simulink library "halin"  (R2021b)
settings: Solver=VariableStepAuto  StartTime=0.0  StopTime=10.0  RelTol=1e-3
undefined symbols (not defined in the file): KHAL_CAN1ABM1E2E_flg, KHAL_CAN1EPB1E2E_flg, KHAL_CAN1EPS1E2E_flg, KHAL_CAN1ESC1E2E_flg, KHAL_CAN1ESC5E2E_flg, KHAL_CAN3BMS1E2E_flg, KHAL_CAN3BMS6E2E_flg, KHAL_CAN3CCU1E2E_flg, KHAL_CAN3CCU2E2E_flg, KHAL_CAN3MCUNF1E2E_flg, KHAL_CAN3MCUNR1E2E_flg, KHAL_CAN3Shifter1E2E_flg, KHAL_CAN3Shifter2E2E_flg, KHAL_CAN6FCM2E2E_flg, KHAL_CAN6FCM4E2E_flg, TRUE
libraries: simulink x645, FVT_lib x212, hcu_lib x59
(part 18 of 23)

== system halin/HAL_IN/CAN1/EPS1/SASSpeedValid ==
  SAS_Speed_Valid : Inport
  UnitConverter : DataTypeConversion  OutDataTypeStr=uint8
  VHAL_SASSpeedValid_flg : Outport
  wires:
  UnitConverter/1 -> VHAL_SASSpeedValid_flg/1
  SAS_Speed_Valid/1 -> UnitConverter/1

== system halin/HAL_IN/CAN1/EPS1/SASV ==
  SAS_V : Inport
  UnitConverter : DataTypeConversion  OutDataTypeStr=uint8
  VHAL_SASV_flg : Outport
  wires:
  UnitConverter/1 -> VHAL_SASV_flg/1
  SAS_V/1 -> UnitConverter/1

== system halin/HAL_IN/CAN1/ESC1/ABSActive ==
  ABS_Active : Inport
  UnitConverter : DataTypeConversion  OutDataTypeStr=uint8
  VHAL_ABSActive_flg : Outport
  wires:
  UnitConverter/1 -> VHAL_ABSActive_flg/1
  ABS_Active/1 -> UnitConverter/1

== system halin/HAL_IN/CAN1/ESC1/ABSFailed ==
  ABS_Failed : Inport
  UnitConverter : DataTypeConversion  OutDataTypeStr=uint8
  VHAL_ABSFailed_flg : Outport
  wires:
  UnitConverter/1 -> VHAL_ABSFailed_flg/1
  ABS_Failed/1 -> UnitConverter/1

== system halin/HAL_IN/CAN1/ESC1/ABSWnlmpSta ==
  ABS_WnlmpSta : Inport
  UnitConverter : DataTypeConversion  OutDataTypeStr=uint8
  VHAL_ABSWnlmpSta_flg : Outport
  wires:
  UnitConverter/1 -> VHAL_ABSWnlmpSta_flg/1
  ABS_WnlmpSta/1 -> UnitConverter/1

== system halin/HAL_IN/CAN1/ESC1/AVHActive ==
  AVH_Active : Inport
  UnitConverter : DataTypeConversion  OutDataTypeStr=uint8
  VHAL_AVHActive_flg : Outport
  wires:
  UnitConverter/1 -> VHAL_AVHActive_flg/1
  AVH_Active/1 -> UnitConverter/1

== system halin/HAL_IN/CAN1/ESC1/AVHFailed ==
  AVH_Failed : Inport
  UnitConverter : DataTypeConversion  OutDataTypeStr=uint8
  VHAL_AVHFailed_flg : Outport
  wires:
  UnitConverter/1 -> VHAL_AVHFailed_flg/1
  AVH_Failed/1 -> UnitConverter/1

== system halin/HAL_IN/CAN1/ESC1/AmberWnlmpSta ==
  Amber_WnlmpSta : Inport
  UnitConverter : DataTypeConversion  OutDataTypeStr=uint8
  VHAL_AmberWnlmpSta_flg : Outport
  wires:
  UnitConverter/1 -> VHAL_AmberWnlmpSta_flg/1
  Amber_WnlmpSta/1 -> UnitConverter/1

== system halin/HAL_IN/CAN1/ESC1/BTCSActive ==
  BTCS_Active : Inport
  UnitConverter : DataTypeConversion  OutDataTypeStr=uint8
  VHAL_BTCSActive_flg : Outport
  wires:
  UnitConverter/1 -> VHAL_BTCSActive_flg/1
  BTCS_Active/1 -> UnitConverter/1

== system halin/HAL_IN/CAN1/ESC1/EBDActive ==
  EBD_Active : Inport
  UnitConverter : DataTypeConversion  OutDataTypeStr=uint8
  VHAL_EBDActive_flg : Outport
  wires:
  UnitConverter/1 -> VHAL_EBDActive_flg/1
  EBD_Active/1 -> UnitConverter/1

== system halin/HAL_IN/CAN1/ESC1/EBDFailed ==
  EBD_Failed : Inport
  UnitConverter : DataTypeConversion  OutDataTypeStr=uint8
  VHAL_EBDFailed_flg : Outport
  wires:
  UnitConverter/1 -> VHAL_EBDFailed_flg/1
  EBD_Failed/1 -> UnitConverter/1

== system halin/HAL_IN/CAN1/ESC1/ESC1CS ==
  ESC1_CS : Inport
  UnitConverter : DataTypeConversion  OutDataTypeStr=uint8
  VHAL_ESC1CS_enum : Outport
  wires:
  UnitConverter/1 -> VHAL_ESC1CS_enum/1
  ESC1_CS/1 -> UnitConverter/1

== system halin/HAL_IN/CAN1/ESC1/ESC1RC ==
  ESC1_RC : Inport
  UnitConverter : DataTypeConversion  OutDataTypeStr=uint8
  VHAL_ESC1RC_enum : Outport
  wires:
  UnitConverter/1 -> VHAL_ESC1RC_enum/1
  ESC1_RC/1 -> UnitConverter/1

== system halin/HAL_IN/CAN1/ESC1/ESCActive ==
  ESC_Active : Inport
  UnitConverter : DataTypeConversion  OutDataTypeStr=uint8
  VHAL_ESCActive_flg : Outport
  wires:
  UnitConverter/1 -> VHAL_ESCActive_flg/1
  ESC_Active/1 -> UnitConverter/1

== system halin/HAL_IN/CAN1/ESC1/ESCBeepReq ==
  ESC_BeepReq : Inport
  UnitConverter : DataTypeConversion  OutDataTypeStr=uint8
  VHAL_ESCBeepReq_flg : Outport
  wires:
  UnitConverter/1 -> VHAL_ESCBeepReq_flg/1
  ESC_BeepReq/1 -> UnitConverter/1

== system halin/HAL_IN/CAN1/ESC1/ESCFailed ==
  ESC_Failed : Inport
  UnitConverter : DataTypeConversion  OutDataTypeStr=uint8
  VHAL_ESCFailed_flg : Outport
  wires:
  UnitConverter/1 -> VHAL_ESCFailed_flg/1
  ESC_Failed/1 -> UnitConverter/1

== system halin/HAL_IN/CAN1/ESC1/ESCOFFStatus ==
  ESC_OFF_Status : Inport
  UnitConverter : DataTypeConversion  OutDataTypeStr=uint8
  VHAL_ESCOFFStatus_enum : Outport
  wires:
  UnitConverter/1 -> VHAL_ESCOFFStatus_enum/1
  ESC_OFF_Status/1 -> UnitConverter/1

== system halin/HAL_IN/CAN1/ESC1/ESCOfflmpSta ==
  ESC_Off_lmpSta : Inport
  UnitConverter : DataTypeConversion  OutDataTypeStr=uint8
  VHAL_ESCOfflmpSta_flg : Outport
  wires:
  UnitConverter/1 -> VHAL_ESCOfflmpSta_flg/1
  ESC_Off_lmpSta/1 -> UnitConverter/1

== system halin/HAL_IN/CAN1/ESC1/ESCWnlmpSta ==
  ESC_WnlmpSta : Inport
  UnitConverter : DataTypeConversion  OutDataTypeStr=uint8
  VHAL_ESCWnlmpSta_enum : Outport
  wires:
  UnitConverter/1 -> VHAL_ESCWnlmpSta_enum/1
  ESC_WnlmpSta/1 -> UnitConverter/1

== system halin/HAL_IN/CAN1/ESC1/ESSActive ==
  ESS_Active : Inport
  UnitConverter : DataTypeConversion  OutDataTypeStr=uint8
  VHAL_ESSActive_flg : Outport
  wires:
  UnitConverter/1 -> VHAL_ESSActive_flg/1
  ESS_Active/1 -> UnitConverter/1

== system halin/HAL_IN/CAN1/ESC1/FrPTCSActive ==
  Fr_PTCS_Active : Inport
  UnitConverter : DataTypeConversion  OutDataTypeStr=uint8
  VHAL_FrPTCSActive_flg : Outport
  wires:
  UnitConverter/1 -> VHAL_FrPTCSActive_flg/1
  Fr_PTCS_Active/1 -> UnitConverter/1

== system halin/HAL_IN/CAN1/ESC1/FrntAxlTrqReqDrv ==
  FrntAxlTrqReq_Drv : Inport
  UnitConverter : DataTypeConversion  OutDataTypeStr=uint16
  convert_in : FVT_lib/hal/convert_in  gain=0.5  offset=-5300
  VHAL_FrntAxlTrqReqDrv_Nm : Outport
  wires:
  convert_in/1 -> VHAL_FrntAxlTrqReqDrv_Nm/1
  UnitConverter/1 -> convert_in/1
  FrntAxlTrqReq_Drv/1 -> UnitConverter/1

== system halin/HAL_IN/CAN1/ESC1/GRADE ==
  GRADE : Inport
  UnitConverter : DataTypeConversion  OutDataTypeStr=uint8
  convert_in : FVT_lib/hal/convert_in  gain=0.35433  offset=-45
  VHAL_GRADE_Deg : Outport
  wires:
  convert_in/1 -> VHAL_GRADE_Deg/1
  UnitConverter/1 -> convert_in/1
  GRADE/1 -> UnitConverter/1

== system halin/HAL_IN/CAN1/ESC1/HBBActive ==
  HBB_Active : Inport
  UnitConverter : DataTypeConversion  OutDataTypeStr=uint8
  VHAL_HBBActive_flg : Outport
  wires:
  UnitConverter/1 -> VHAL_HBBActive_flg/1
  HBB_Active/1 -> UnitConverter/1

== system halin/HAL_IN/CAN1/ESC1/HBBFailed ==
  HBB_Failed : Inport
  UnitConverter : DataTypeConversion  OutDataTypeStr=uint8
  VHAL_HBBFailed_flg : Outport
  wires:
  UnitConverter/1 -> VHAL_HBBFailed_flg/1
  HBB_Failed/1 -> UnitConverter/1

== system halin/HAL_IN/CAN1/ESC1/HDDActive ==
  HDD_Active : Inport
  UnitConverter : DataTypeConversion  OutDataTypeStr=uint8
  VHAL_HDDActive_flg : Outport
  wires:
  UnitConverter/1 -> VHAL_HDDActive_flg/1
  HDD_Active/1 -> UnitConverter/1

== system halin/HAL_IN/CAN1/ESC1/HDDFailed ==
  HDD_Failed : Inport
  UnitConverter : DataTypeConversion  OutDataTypeStr=uint8
  VHAL_HDDFailed_flg : Outport
  wires:
  UnitConverter/1 -> VHAL_HDDFailed_flg/1
  HDD_Failed/1 -> UnitConverter/1

== system halin/HAL_IN/CAN1/ESC1/HSAActive ==
  HSA_Active : Inport
  UnitConverter : DataTypeConversion  OutDataTypeStr=uint8
  VHAL_HSAActive_flg : Outport
  wires:
  UnitConverter/1 -> VHAL_HSAActive_flg/1
  HSA_Active/1 -> UnitConverter/1

== system halin/HAL_IN/CAN1/ESC1/HSAFailed ==
  HSA_Failed : Inport
  UnitConverter : DataTypeConversion  OutDataTypeStr=uint8
  VHAL_HSAFailed_flg : Outport
  wires:
  UnitConverter/1 -> VHAL_HSAFailed_flg/1
  HSA_Failed/1 -> UnitConverter/1

== system halin/HAL_IN/CAN1/ESC1/LFPulseCount ==
  LF_PulseCount : Inport
  UnitConverter : DataTypeConversion  OutDataTypeStr=uint8
  VHAL_LFPulseCount_enum : Outport
  wires:
  UnitConverter/1 -> VHAL_LFPulseCount_enum/1
  LF_PulseCount/1 -> UnitConverter/1

== system halin/HAL_IN/CAN1/ESC1/LFPulseCountV ==
  LF_PulseCount_V : Inport
  UnitConverter : DataTypeConversion  OutDataTypeStr=uint8
  VHAL_LFPulseCountV_flg : Outport
  wires:
  UnitConverter/1 -> VHAL_LFPulseCountV_flg/1
  LF_PulseCount_V/1 -> UnitConverter/1

== system halin/HAL_IN/CAN1/ESC1/LFRawWhlSpeed ==
  LF_RawWhlSpeed : Inport
  UnitConverter : DataTypeConversion  OutDataTypeStr=uint16
  convert_in : FVT_lib/hal/convert_in  gain=0.0625  offset=0
  VHAL_LFRawWhlSpeed_kph : Outport
  wires:
  convert_in/1 -> VHAL_LFRawWhlSpeed_kph/1
  UnitConverter/1 -> convert_in/1
  LF_RawWhlSpeed/1 -> UnitConverter/1

== system halin/HAL_IN/CAN1/ESC1/LFRawWhlSpeedV ==
  LF_RawWhlSpeed_V : Inport
  UnitConverter : DataTypeConversion  OutDataTypeStr=uint8
  VHAL_LFRawWhlSpeedV_flg : Outport
  wires:
  UnitConverter/1 -> VHAL_LFRawWhlSpeedV_flg/1
  LF_RawWhlSpeed_V/1 -> UnitConverter/1

== system halin/HAL_IN/CAN1/ESC1/LFWhlRotDir ==
  LF_WhlRotDir : Inport
  UnitConverter : DataTypeConversion  OutDataTypeStr=uint8
  VHAL_LFWhlRotDir_enum : Outport
  wires:
  UnitConverter/1 -> VHAL_LFWhlRotDir_enum/1
  LF_WhlRotDir/1 -> UnitConverter/1

== system halin/HAL_IN/CAN1/ESC1/LRPulseCount ==
  LR_PulseCount : Inport
  UnitConverter : DataTypeConversion  OutDataTypeStr=uint8
  VHAL_LRPulseCount_enum : Outport
  wires:
  UnitConverter/1 -> VHAL_LRPulseCount_enum/1
  LR_PulseCount/1 -> UnitConverter/1

== system halin/HAL_IN/CAN1/ESC1/LRPulseCountV ==
  LR_PulseCount_V : Inport
  UnitConverter : DataTypeConversion  OutDataTypeStr=uint8
  VHAL_LRPulseCountV_flg : Outport
  wires:
  UnitConverter/1 -> VHAL_LRPulseCountV_flg/1
  LR_PulseCount_V/1 -> UnitConverter/1

== system halin/HAL_IN/CAN1/ESC1/LRRawWhlSpeed ==
  LR_RawWhlSpeed : Inport
  UnitConverter : DataTypeConversion  OutDataTypeStr=uint16
  convert_in : FVT_lib/hal/convert_in  gain=0.0625  offset=0
  VHAL_LRRawWhlSpeed_kph : Outport
  wires:
  convert_in/1 -> VHAL_LRRawWhlSpeed_kph/1
  UnitConverter/1 -> convert_in/1
  LR_RawWhlSpeed/1 -> UnitConverter/1

== system halin/HAL_IN/CAN1/ESC1/LRRawWhlSpeedV ==
  LR_RawWhlSpeed_V : Inport
  UnitConverter : DataTypeConversion  OutDataTypeStr=uint8
  VHAL_LRRawWhlSpeedV_flg : Outport
  wires:
  UnitConverter/1 -> VHAL_LRRawWhlSpeedV_flg/1
  LR_RawWhlSpeed_V/1 -> UnitConverter/1

== system halin/HAL_IN/CAN1/ESC1/LRWhlRotDir ==
  LR_WhlRotDir : Inport
  UnitConverter : DataTypeConversion  OutDataTypeStr=uint8
  VHAL_LRWhlRotDir_enum : Outport
  wires:
  UnitConverter/1 -> VHAL_LRWhlRotDir_enum/1
  LR_WhlRotDir/1 -> UnitConverter/1

== system halin/HAL_IN/CAN1/ESC1/PBAActive ==
  PBA_Active : Inport
  UnitConverter : DataTypeConversion  OutDataTypeStr=uint8
  VHAL_PBAActive_flg : Outport
  wires:
  UnitConverter/1 -> VHAL_PBAActive_flg/1
  PBA_Active/1 -> UnitConverter/1

== system halin/HAL_IN/CAN1/ESC1/PBAFailed ==
  PBA_Failed : Inport
  UnitConverter : DataTypeConversion  OutDataTypeStr=uint8
  VHAL_PBAFailed_flg : Outport
  wires:
  UnitConverter/1 -> VHAL_PBAFailed_flg/1
  PBA_Failed/1 -> UnitConverter/1

== system halin/HAL_IN/CAN1/ESC1/RFPulseCount ==
  RF_PulseCount : Inport
  UnitConverter : DataTypeConversion  OutDataTypeStr=uint8
  VHAL_RFPulseCount_enum : Outport
  wires:
  UnitConverter/1 -> VHAL_RFPulseCount_enum/1
  RF_PulseCount/1 -> UnitConverter/1

== system halin/HAL_IN/CAN1/ESC1/RFPulseCountV ==
  RF_PulseCount_V : Inport
  UnitConverter : DataTypeConversion  OutDataTypeStr=uint8
  VHAL_RFPulseCountV_flg : Outport
  wires:
  UnitConverter/1 -> VHAL_RFPulseCountV_flg/1
  RF_PulseCount_V/1 -> UnitConverter/1

== system halin/HAL_IN/CAN1/ESC1/RFRawWhlSpeed ==
  RF_RawWhlSpeed : Inport
  UnitConverter : DataTypeConversion  OutDataTypeStr=uint16
  convert_in : FVT_lib/hal/convert_in  gain=0.0625  offset=0
  VHAL_RFRawWhlSpeed_kph : Outport
  wires:
  convert_in/1 -> VHAL_RFRawWhlSpeed_kph/1
  UnitConverter/1 -> convert_in/1
  RF_RawWhlSpeed/1 -> UnitConverter/1

== system halin/HAL_IN/CAN1/ESC1/RFRawWhlSpeedV ==
  RF_RawWhlSpeed_V : Inport
  UnitConverter : DataTypeConversion  OutDataTypeStr=uint8
  VHAL_RFRawWhlSpeedV_flg : Outport
  wires:
  UnitConverter/1 -> VHAL_RFRawWhlSpeedV_flg/1
  RF_RawWhlSpeed_V/1 -> UnitConverter/1

== system halin/HAL_IN/CAN1/ESC1/RFWhlRotDir ==
  RF_WhlRotDir : Inport
  UnitConverter : DataTypeConversion  OutDataTypeStr=uint8
  VHAL_RFWhlRotDir_enum : Outport
  wires:
  UnitConverter/1 -> VHAL_RFWhlRotDir_enum/1
  RF_WhlRotDir/1 -> UnitConverter/1

== system halin/HAL_IN/CAN1/ESC1/RRPulseCount ==
  RR_PulseCount : Inport
  UnitConverter : DataTypeConversion  OutDataTypeStr=uint8
  VHAL_RRPulseCount_enum : Outport
  wires:
  UnitConverter/1 -> VHAL_RRPulseCount_enum/1
  RR_PulseCount/1 -> UnitConverter/1

== system halin/HAL_IN/CAN1/ESC1/RRPulseCountV ==
  RR_PulseCount_V : Inport
  UnitConverter : DataTypeConversion  OutDataTypeStr=uint8
  VHAL_RRPulseCountV_flg : Outport
  wires:
  UnitConverter/1 -> VHAL_RRPulseCountV_flg/1
  RR_PulseCount_V/1 -> UnitConverter/1

== system halin/HAL_IN/CAN1/ESC1/RRRawWhlSpeed ==
  RR_RawWhlSpeed : Inport
  UnitConverter : DataTypeConversion  OutDataTypeStr=uint16
  convert_in : FVT_lib/hal/convert_in  gain=0.0625  offset=0
  VHAL_RRRawWhlSpeed_kph : Outport
  wires:
  convert_in/1 -> VHAL_RRRawWhlSpeed_kph/1
  UnitConverter/1 -> convert_in/1
  RR_RawWhlSpeed/1 -> UnitConverter/1

== system halin/HAL_IN/CAN1/ESC1/RRRawWhlSpeedV ==
  RR_RawWhlSpeed_V : Inport
  UnitConverter : DataTypeConversion  OutDataTypeStr=uint8
  VHAL_RRRawWhlSpeedV_flg : Outport
  wires:
  UnitConverter/1 -> VHAL_RRRawWhlSpeedV_flg/1
  RR_RawWhlSpeed_V/1 -> UnitConverter/1

== system halin/HAL_IN/CAN1/ESC1/RRWhlRotDir ==
  RR_WhlRotDir : Inport
  UnitConverter : DataTypeConversion  OutDataTypeStr=uint8
  VHAL_RRWhlRotDir_enum : Outport
  wires:
  UnitConverter/1 -> VHAL_RRWhlRotDir_enum/1
  RR_WhlRotDir/1 -> UnitConverter/1

== system halin/HAL_IN/CAN1/ESC1/RearAxlTrqReqDrv ==
  RearAxlTrqReq_Drv : Inport
  UnitConverter : DataTypeConversion  OutDataTypeStr=uint16
  convert_in : FVT_lib/hal/convert_in  gain=0.5  offset=-5300
  VHAL_RearAxlTrqReqDrv_Nm : Outport
  wires:
  convert_in/1 -> VHAL_RearAxlTrqReqDrv_Nm/1
  UnitConverter/1 -> convert_in/1
  RearAxlTrqReq_Drv/1 -> UnitConverter/1

== system halin/HAL_IN/CAN1/ESC1/RedWnlmpSta ==
  Red_WnlmpSta : Inport
  UnitConverter : DataTypeConversion  OutDataTypeStr=uint8
  VHAL_RedWnlmpSta_flg : Outport
  wires:
  UnitConverter/1 -> VHAL_RedWnlmpSta_flg/1
  Red_WnlmpSta/1 -> UnitConverter/1

== system halin/HAL_IN/CAN1/ESC1/RrPTCSActive ==
  Rr_PTCS_Active : Inport
  UnitConverter : DataTypeConversion  OutDataTypeStr=uint8
  VHAL_RrPTCSActive_flg : Outport
  wires:
  UnitConverter/1 -> VHAL_RrPTCSActive_flg/1
  Rr_PTCS_Active/1 -> UnitConverter/1

== system halin/HAL_IN/CAN1/ESC1/TCSActive ==
  TCS_Active : Inport
  UnitConverter : DataTypeConversion  OutDataTypeStr=uint8
  VHAL_TCSActive_flg : Outport
  wires:
  UnitConverter/1 -> VHAL_TCSActive_flg/1
  TCS_Active/1 -> UnitConverter/1

== system halin/HAL_IN/CAN1/ESC1/TCSFailed ==
  TCS_Failed : Inport
  UnitConverter : DataTypeConversion  OutDataTypeStr=uint8
  VHAL_TCSFailed_flg : Outport
  wires:
  UnitConverter/1 -> VHAL_TCSFailed_flg/1
  TCS_Failed/1 -> UnitConverter/1

== system halin/HAL_IN/CAN1/ESC1/VehSpeed ==
  VehSpeed : Inport
  UnitConverter : DataTypeConversion  OutDataTypeStr=uint16
  convert_in : FVT_lib/hal/convert_in  gain=0.125  offset=0
  VHAL_VehSpeed_kph : Outport
  wires:
  convert_in/1 -> VHAL_VehSpeed_kph/1
  UnitConverter/1 -> convert_in/1
  VehSpeed/1 -> UnitConverter/1

== system halin/HAL_IN/CAN1/ESC5/ACCAvail ==
  ACCAvail : Inport
  UnitConverter : DataTypeConversion  OutDataTypeStr=uint8
  VHAL_ACCAvail_flg : Outport
  wires:
  UnitConverter/1 -> VHAL_ACCAvail_flg/1
  ACCAvail/1 -> UnitConverter/1

== system halin/HAL_IN/CAN1/ESC5/AEBAvail ==
  AEBAvail : Inport
  UnitConverter : DataTypeConversion  OutDataTypeStr=uint8
  VHAL_AEBAvail_flg : Outport
  wires:
  UnitConverter/1 -> VHAL_AEBAvail_flg/1
  AEBAvail/1 -> UnitConverter/1

== system halin/HAL_IN/CAN1/ESC5/ActBrkLampSta ==
  ActBrkLamp_Sta : Inport
  UnitConverter : DataTypeConversion  OutDataTypeStr=uint8
  VHAL_ActBrkLampSta_flg : Outport
  wires:
  UnitConverter/1 -> VHAL_ActBrkLampSta_flg/1
  ActBrkLamp_Sta/1 -> UnitConverter/1

== system halin/HAL_IN/CAN1/ESC5/BrkDiscTempSta ==
  BrkDiscTempSta : Inport
  UnitConverter : DataTypeConversion  OutDataTypeStr=uint8
  VHAL_BrkDiscTempSta_flg : Outport
  wires:
  UnitConverter/1 -> VHAL_BrkDiscTempSta_flg/1
  BrkDiscTempSta/1 -> UnitConverter/1

== system halin/HAL_IN/CAN1/ESC5/BrkPedalPos ==
  BrkPedalPos : Inport
  UnitConverter : DataTypeConversion  OutDataTypeStr=uint8
  convert_in : FVT_lib/hal/convert_in  gain=0.4  offset=0
  VHAL_BrkPedalPos_pct : Outport
  wires:
  convert_in/1 -> VHAL_BrkPedalPos_pct/1
  UnitConverter/1 -> convert_in/1
  BrkPedalPos/1 -> UnitConverter/1

== system halin/HAL_IN/CAN1/ESC5/BrkPedalPosSta ==
  BrkPedalPos_Sta : Inport
  UnitConverter : DataTypeConversion  OutDataTypeStr=uint8
  VHAL_BrkPedalPosSta_flg : Outport
  wires:
  UnitConverter/1 -> VHAL_BrkPedalPosSta_flg/1
  BrkPedalPos_Sta/1 -> UnitConverter/1

== system halin/HAL_IN/CAN1/ESC5/BrkSwSta ==
  BrkSw_Sta : Inport
  UnitConverter : DataTypeConversion  OutDataTypeStr=uint8
  VHAL_BrkSwSta_flg : Outport
  wires:
  UnitConverter/1 -> VHAL_BrkSwSta_flg/1
  BrkSw_Sta/1 -> UnitConverter/1

== system halin/HAL_IN/CAN1/ESC5/BrkSwV ==
  BrkSw_V : Inport
  UnitConverter : DataTypeConversion  OutDataTypeStr=uint8
  VHAL_BrkSwV_flg : Outport
  wires:
  UnitConverter/1 -> VHAL_BrkSwV_flg/1
  BrkSw_V/1 -> UnitConverter/1

== system halin/HAL_IN/CAN1/ESC5/ESC5CS ==
  ESC5_CS : Inport
  UnitConverter : DataTypeConversion  OutDataTypeStr=uint8
  VHAL_ESC5CS_enum : Outport
  wires:
  UnitConverter/1 -> VHAL_ESC5CS_enum/1
  ESC5_CS/1 -> UnitConverter/1

== system halin/HAL_IN/CAN1/ESC5/ESC5RC ==
  ESC5_RC : Inport
  UnitConverter : DataTypeConversion  OutDataTypeStr=uint8
  VHAL_ESC5RC_enum : Outport
  wires:
  UnitConverter/1 -> VHAL_ESC5RC_enum/1
  ESC5_RC/1 -> UnitConverter/1

== system halin/HAL_IN/CAN1/ESC5/ESCADASSta ==
  ESC_ADAS_Sta : Inport
  UnitConverter : DataTypeConversion  OutDataTypeStr=uint8
  VHAL_ESCADASSta_enum : Outport
  wires:
  UnitConverter/1 -> VHAL_ESCADASSta_enum/1
  ESC_ADAS_Sta/1 -> UnitConverter/1

== system halin/HAL_IN/CAN1/ESC5/ESCAPSSta ==
  ESC_APS_Sta : Inport
  UnitConverter : DataTypeConversion  OutDataTypeStr=uint8
  VHAL_ESCAPSSta_enum : Outport
  wires:
  UnitConverter/1 -> VHAL_ESCAPSSta_enum/1
  ESC_APS_Sta/1 -> UnitConverter/1

== system halin/HAL_IN/CAN1/ESC5/ESCStandstill ==
  ESC_Standstill : Inport
  UnitConverter : DataTypeConversion  OutDataTypeStr=uint8
  VHAL_ESCStandstill_flg : Outport
  wires:
  UnitConverter/1 -> VHAL_ESCStandstill_flg/1
  ESC_Standstill/1 -> UnitConverter/1

== system halin/HAL_IN/CAN1/ESC5/FrRBCActive ==
  Fr_RBC_Active : Inport
  UnitConverter : DataTypeConversion  OutDataTypeStr=uint8
  VHAL_FrRBCActive_flg : Outport
  wires:
  UnitConverter/1 -> VHAL_FrRBCActive_flg/1
  Fr_RBC_Active/1 -> UnitConverter/1

== system halin/HAL_IN/CAN1/ESC5/FrntAxlTrqReqBrk ==
  FrntAxlTrqReq_Brk : Inport
  UnitConverter : DataTypeConversion  OutDataTypeStr=uint16
  convert_in : FVT_lib/hal/convert_in  gain=0.5  offset=-5300
  VHAL_FrntAxlTrqReqBrk_Nm : Outport
  wires:
  convert_in/1 -> VHAL_FrntAxlTrqReqBrk_Nm/1
  UnitConverter/1 -> convert_in/1
  FrntAxlTrqReq_Brk/1 -> UnitConverter/1

== system halin/HAL_IN/CAN1/ESC5/LatAccel ==
  LatAccel : Inport
  UnitConverter : DataTypeConversion  OutDataTypeStr=uint8
  convert_in : FVT_lib/hal/convert_in  gain=0.01  offset=-1.27
  VHAL_LatAccel_Gps : Outport
  wires:
  convert_in/1 -> VHAL_LatAccel_Gps/1
  UnitConverter/1 -> convert_in/1
  LatAccel/1 -> UnitConverter/1

== system halin/HAL_IN/CAN1/ESC5/LatAccelV ==
  LatAccel_V : Inport
  UnitConverter : DataTypeConversion  OutDataTypeStr=uint8
  VHAL_LatAccelV_flg : Outport
  wires:
  UnitConverter/1 -> VHAL_LatAccelV_flg/1
  LatAccel_V/1 -> UnitConverter/1

== system halin/HAL_IN/CAN1/ESC5/LongAccel ==
  LongAccel : Inport
  UnitConverter : DataTypeConversion  OutDataTypeStr=uint8
  convert_in : FVT_lib/hal/convert_in  gain=0.01  offset=-1.27
  VHAL_LongAccel_Gps : Outport
  wires:
  convert_in/1 -> VHAL_LongAccel_Gps/1
  UnitConverter/1 -> convert_in/1
  LongAccel/1 -> UnitConverter/1

== system halin/HAL_IN/CAN1/ESC5/LongAccelV ==
  LongAccel_V : Inport
  UnitConverter : DataTypeConversion  OutDataTypeStr=uint8
  VHAL_LongAccelV_flg : Outport
  wires:
  UnitConverter/1 -> VHAL_LongAccelV_flg/1
  LongAccel_V/1 -> UnitConverter/1

== system halin/HAL_IN/CAN1/ESC5/MCPressure ==
  MCPressure : Inport
  UnitConverter : DataTypeConversion  OutDataTypeStr=uint16
  convert_in : FVT_lib/hal/convert_in  gain=0.1  offset=-9.7
  VHAL_MCPressure_bar : Outport
  wires:
  convert_in/1 -> VHAL_MCPressure_bar/1
  UnitConverter/1 -> convert_in/1
  MCPressure/1 -> UnitConverter/1

== system halin/HAL_IN/CAN1/ESC5/MCPressureV ==
  MCPressure_V : Inport
  UnitConverter : DataTypeConversion  OutDataTypeStr=uint8
  VHAL_MCPressureV_flg : Outport
  wires:
  UnitConverter/1 -> VHAL_MCPressureV_flg/1
  MCPressure_V/1 -> UnitConverter/1

== system halin/HAL_IN/CAN1/ESC5/MeterIndVehSpeed ==
  Meter_Ind_VehSpeed : Inport
  UnitConverter : DataTypeConversion  OutDataTypeStr=uint16
  convert_in : FVT_lib/hal/convert_in  gain=0.125  offset=0
  VHAL_MeterIndVehSpeed_kph : Outport
  wires:
  convert_in/1 -> VHAL_MeterIndVehSpeed_kph/1
  UnitConverter/1 -> convert_in/1
  Meter_Ind_VehSpeed/1 -> UnitConverter/1

== system halin/HAL_IN/CAN1/ESC5/RDCActive ==
  RDC_Active : Inport
  UnitConverter : DataTypeConversion  OutDataTypeStr=uint8
  VHAL_RDCActive_enum : Outport
  wires:
  UnitConverter/1 -> VHAL_RDCActive_enum/1
  RDC_Active/1 -> UnitConverter/1

== system halin/HAL_IN/CAN1/ESC5/RearAxlTrqReqBrk ==
  RearAxlTrqReq_Brk : Inport
  UnitConverter : DataTypeConversion  OutDataTypeStr=uint16
  convert_in : FVT_lib/hal/convert_in  gain=0.5  offset=-5300
  VHAL_RearAxlTrqReqBrk_Nm : Outport
  wires:
  convert_in/1 -> VHAL_RearAxlTrqReqBrk_Nm/1
  UnitConverter/1 -> convert_in/1
  RearAxlTrqReq_Brk/1 -> UnitConverter/1

== system halin/HAL_IN/CAN1/ESC5/RrRBCActive ==
  Rr_RBC_Active : Inport
  UnitConverter : DataTypeConversion  OutDataTypeStr=uint8
  VHAL_RrRBCActive_flg : Outport
  wires:
  UnitConverter/1 -> VHAL_RrRBCActive_flg/1
  Rr_RBC_Active/1 -> UnitConverter/1

== system halin/HAL_IN/CAN1/ESC5/YawRate ==
  YawRate : Inport
  UnitConverter : DataTypeConversion  OutDataTypeStr=uint16
  convert_in : FVT_lib/hal/convert_in  gain=0.1  offset=-100
  VHAL_YawRate_degps : Outport
  wires:
  convert_in/1 -> VHAL_YawRate_degps/1
  UnitConverter/1 -> convert_in/1
  YawRate/1 -> UnitConverter/1

== system halin/HAL_IN/CAN1/ESC5/YawRateV ==
  YawRate_V : Inport
  UnitConverter : DataTypeConversion  OutDataTypeStr=uint8
  VHAL_YawRateV_flg : Outport
  wires:
  UnitConverter/1 -> VHAL_YawRateV_flg/1
  YawRate_V/1 -> UnitConverter/1

== system halin/HAL_IN/CAN1/eBST1/LowBrakeFluidSta ==
  LowBrakeFluid_Sta : Inport
  UnitConverter : DataTypeConversion  OutDataTypeStr=uint8
  VHAL_LowBrakeFluidSta_flg : Outport
  wires:
  UnitConverter/1 -> VHAL_LowBrakeFluidSta_flg/1
  LowBrakeFluid_Sta/1 -> UnitConverter/1

== system halin/HAL_IN/CAN1/eBST1/eBSTAmberWnlmpSta ==
  eBST_AmberWnlmpSta : Inport
  UnitConverter : DataTypeConversion  OutDataTypeStr=uint8
  VHAL_eBSTAmberWnlmpSta_flg : Outport
  wires:
  UnitConverter/1 -> VHAL_eBSTAmberWnlmpSta_flg/1
  eBST_AmberWnlmpSta/1 -> UnitConverter/1

== system halin/HAL_IN/CAN1/eBST1/eBSTBeepReq ==
  eBST_BeepReq : Inport
  UnitConverter : DataTypeConversion  OutDataTypeStr=uint8
  VHAL_eBSTBeepReq_flg : Outport
  wires:
  UnitConverter/1 -> VHAL_eBSTBeepReq_flg/1
  eBST_BeepReq/1 -> UnitConverter/1

== system halin/HAL_IN/CAN1/eBST1/eBSTRedWnlmpSta ==
  eBST_RedWnlmpSta : Inport
  UnitConverter : DataTypeConversion  OutDataTypeStr=uint8
  VHAL_eBSTRedWnlmpSta_flg : Outport
  wires:
  UnitConverter/1 -> VHAL_eBSTRedWnlmpSta_flg/1
  eBST_RedWnlmpSta/1 -> UnitConverter/1

== system halin/HAL_IN/CAN2/HMI1/HMIACAirIntMCmd ==
  HMI_ACAirIntM_Cmd : Inport
  UnitConverter : DataTypeConversion  OutDataTypeStr=uint8
  VHAL_HMIACAirIntMCmd_flg : Outport
  wires:
  UnitConverter/1 -> VHAL_HMIACAirIntMCmd_flg/1
  HMI_ACAirIntM_Cmd/1 -> UnitConverter/1

== system halin/HAL_IN/CAN2/HMI1/HMIACAirIntPCmd ==
  HMI_ACAirIntP_Cmd : Inport
  UnitConverter : DataTypeConversion  OutDataTypeStr=uint8
  VHAL_HMIACAirIntPCmd_flg : Outport
  wires:
  UnitConverter/1 -> VHAL_HMIACAirIntPCmd_flg/1
  HMI_ACAirIntP_Cmd/1 -> UnitConverter/1

== system halin/HAL_IN/CAN2/HMI1/HMIACAutoBtnCmd ==
  HMI_ACAutoBtn_Cmd : Inport
  UnitConverter : DataTypeConversion  OutDataTypeStr=uint8
  VHAL_HMIACAutoBtnCmd_flg : Outport
  wires:
  UnitConverter/1 -> VHAL_HMIACAutoBtnCmd_flg/1
  HMI_ACAutoBtn_Cmd/1 -> UnitConverter/1

== system halin/HAL_IN/CAN2/HMI1/HMIACBtnCmd ==
  HMI_ACBtn_Cmd : Inport
  UnitConverter : DataTypeConversion  OutDataTypeStr=uint8
  VHAL_HMIACBtnCmd_flg : Outport
  wires:
  UnitConverter/1 -> VHAL_HMIACBtnCmd_flg/1
  HMI_ACBtn_Cmd/1 -> UnitConverter/1

== system halin/HAL_IN/CAN2/HMI1/HMIACFrDefogBtnCmd ==
  HMI_ACFrDefogBtn_Cmd : Inport
  UnitConverter : DataTypeConversion  OutDataTypeStr=uint8
  VHAL_HMIACFrDefogBtnCmd_flg : Outport
  wires:
  UnitConverter/1 -> VHAL_HMIACFrDefogBtnCmd_flg/1
  HMI_ACFrDefogBtn_Cmd/1 -> UnitConverter/1

== system halin/HAL_IN/CAN2/HMI1/HMIACRecycleBtnCmd ==
  HMI_ACRecycleBtn_Cmd : Inport
  UnitConverter : DataTypeConversion  OutDataTypeStr=uint8
  VHAL_HMIACRecycleBtnCmd_flg : Outport
  wires:
  UnitConverter/1 -> VHAL_HMIACRecycleBtnCmd_flg/1
  HMI_ACRecycleBtn_Cmd/1 -> UnitConverter/1

== system halin/HAL_IN/CAN2/HMI1/HMIACWindDirMCmd ==
  HMI_ACWindDirM_Cmd : Inport
  UnitConverter : DataTypeConversion  OutDataTypeStr=uint8
  VHAL_HMIACWindDirMCmd_flg : Outport
  wires:
  UnitConverter/1 -> VHAL_HMIACWindDirMCmd_flg/1
  HMI_ACWindDirM_Cmd/1 -> UnitConverter/1

== system halin/HAL_IN/CAN2/HMI1/HMIACWindDirPCmd ==
  HMI_ACWindDirP_Cmd : Inport
  UnitConverter : DataTypeConversion  OutDataTypeStr=uint8
  VHAL_HMIACWindDirPCmd_flg : Outport
  wires:
  UnitConverter/1 -> VHAL_HMIACWindDirPCmd_flg/1
  HMI_ACWindDirP_Cmd/1 -> UnitConverter/1

== system halin/HAL_IN/CAN2/HMI1/HMIAutoInterLightCmd ==
  HMI_AutoInterLight_Cmd : Inport
  UnitConverter : DataTypeConversion  OutDataTypeStr=uint8
  VHAL_HMIAutoInterLightCmd_flg : Outport
  wires:
  UnitConverter/1 -> VHAL_HMIAutoInterLightCmd_flg/1
  HMI_AutoInterLight_Cmd/1 -> UnitConverter/1

== system halin/HAL_IN/CAN2/HMI1/HMIBCMPostDefogBtnCmd ==
  HMI_BCMPostDefogBtn_Cmd : Inport
  UnitConverter : DataTypeConversion  OutDataTypeStr=uint8
  VHAL_HMIBCMPostDefogBtnCmd_flg : Outport
  wires:
  UnitConverter/1 -> VHAL_HMIBCMPostDefogBtnCmd_flg/1
  HMI_BCMPostDefogBtn_Cmd/1 -> UnitConverter/1

== system halin/HAL_IN/CAN2/HMI1/HMIZ1SetTMCmd ==
  HMI_Z1SetTM_Cmd : Inport
  UnitConverter : DataTypeConversion  OutDataTypeStr=uint8
  VHAL_HMIZ1SetTMCmd_flg : Outport
  wires:
  UnitConverter/1 -> VHAL_HMIZ1SetTMCmd_flg/1
  HMI_Z1SetTM_Cmd/1 -> UnitConverter/1

== system halin/HAL_IN/CAN2/HMI1/HMIZ1SetTPCmd ==
  HMI_Z1SetTP_Cmd : Inport
  UnitConverter : DataTypeConversion  OutDataTypeStr=uint8
  VHAL_HMIZ1SetTPCmd_flg : Outport
  wires:
  UnitConverter/1 -> VHAL_HMIZ1SetTPCmd_flg/1
  HMI_Z1SetTP_Cmd/1 -> UnitConverter/1

== system halin/HAL_IN/CAN2/HMI1/HMIZ2SetTMCmd ==
  HMI_Z2SetTM_Cmd : Inport
  UnitConverter : DataTypeConversion  OutDataTypeStr=uint8
  VHAL_HMIZ2SetTMCmd_flg : Outport
  wires:
  UnitConverter/1 -> VHAL_HMIZ2SetTMCmd_flg/1
  HMI_Z2SetTM_Cmd/1 -> UnitConverter/1

== system halin/HAL_IN/CAN2/HMI1/HMIZ2SetTPCmd ==
  HMI_Z2SetTP_Cmd : Inport
  UnitConverter : DataTypeConversion  OutDataTypeStr=uint8
  VHAL_HMIZ2SetTPCmd_flg : Outport
  wires:
  UnitConverter/1 -> VHAL_HMIZ2SetTPCmd_flg/1
  HMI_Z2SetTP_Cmd/1 -> UnitConverter/1

== system halin/HAL_IN/CAN2/IVI1/AmbLighLowBatAlertSW ==
  AmbLigh_LowBatAlert_SW : Inport
  UnitConverter : DataTypeConversion  OutDataTypeStr=uint8
  VHAL_AmbLighLowBatAlertSW_flg : Outport
  wires:
  UnitConverter/1 -> VHAL_AmbLighLowBatAlertSW_flg/1
  AmbLigh_LowBatAlert_SW/1 -> UnitConverter/1

== system halin/HAL_IN/CAN2/IVI1/AmbLighSafetyAlertSW ==
  AmbLigh_SafetyAlert_SW : Inport
  UnitConverter : DataTypeConversion  OutDataTypeStr=uint8
  VHAL_AmbLighSafetyAlertSW_flg : Outport
  wires:
  UnitConverter/1 -> VHAL_AmbLighSafetyAlertSW_flg/1
  AmbLigh_SafetyAlert_SW/1 -> UnitConverter/1

== system halin/HAL_IN/CAN2/IVI1/AmbLightBrightnessSet ==
  AmbLightBrightnessSet : Inport
  UnitConverter : DataTypeConversion  OutDataTypeStr=uint8
  VHAL_AmbLightBrightnessSet_enum : Outport
  wires:
  UnitConverter/1 -> VHAL_AmbLightBrightnessSet_enum/1
  AmbLightBrightnessSet/1 -> UnitConverter/1

== system halin/HAL_IN/CAN2/IVI1/AmbLightColorSet ==
  AmbLightColorSet : Inport
  UnitConverter : DataTypeConversion  OutDataTypeStr=uint8
  VHAL_AmbLightColorSet_enum : Outport
  wires:
  UnitConverter/1 -> VHAL_AmbLightColorSet_enum/1
  AmbLightColorSet/1 -> UnitConverter/1

== system halin/HAL_IN/CAN2/IVI1/AmbLightDimInDarkSW ==
  AmbLight_DimInDark_SW : Inport
  UnitConverter : DataTypeConversion  OutDataTypeStr=uint8
  VHAL_AmbLightDimInDarkSW_flg : Outport
  wires:
  UnitConverter/1 -> VHAL_AmbLightDimInDarkSW_flg/1
  AmbLight_DimInDark_SW/1 -> UnitConverter/1

== system halin/HAL_IN/CAN2/IVI1/AmbLightSW ==
  AmbLight_SW : Inport
  UnitConverter : DataTypeConversion  OutDataTypeStr=uint8
  VHAL_AmbLightSW_flg : Outport
  wires:
  UnitConverter/1 -> VHAL_AmbLightSW_flg/1
  AmbLight_SW/1 -> UnitConverter/1

== system halin/HAL_IN/CAN2/IVI1/AmbLightWlcmLightSW ==
  AmbLight_WlcmLight_SW : Inport
  UnitConverter : DataTypeConversion  OutDataTypeStr=uint8
  VHAL_AmbLightWlcmLightSW_flg : Outport
  wires:
  UnitConverter/1 -> VHAL_AmbLightWlcmLightSW_flg/1
  AmbLight_WlcmLight_SW/1 -> UnitConverter/1

== system halin/HAL_IN/CAN2/IVI1/FCPFrEvtBtnACMaxReq ==
  FCP_FrEvt_BtnACMaxReq : Inport
  UnitConverter : DataTypeConversion  OutDataTypeStr=uint8
  VHAL_FCPFrEvtBtnACMaxReq_flg : Outport
  wires:
  UnitConverter/1 -> VHAL_FCPFrEvtBtnACMaxReq_flg/1
  FCP_FrEvt_BtnACMaxReq/1 -> UnitConverter/1

== system halin/HAL_IN/CAN2/IVI1/FCPFrEvtBtnACReq ==
  FCP_FrEvt_BtnACReq : Inport
  UnitConverter : DataTypeConversion  OutDataTypeStr=uint8
  VHAL_FCPFrEvtBtnACReq_flg : Outport
  wires:
  UnitConverter/1 -> VHAL_FCPFrEvtBtnACReq_flg/1
  FCP_FrEvt_BtnACReq/1 -> UnitConverter/1

== system halin/HAL_IN/CAN2/IVI1/FCPFrEvtBtnAutoReq ==
  FCP_FrEvt_BtnAutoReq : Inport
  UnitConverter : DataTypeConversion  OutDataTypeStr=uint8
  VHAL_FCPFrEvtBtnAutoReq_flg : Outport
  wires:
  UnitConverter/1 -> VHAL_FCPFrEvtBtnAutoReq_flg/1
  FCP_FrEvt_BtnAutoReq/1 -> UnitConverter/1

== system halin/HAL_IN/CAN2/IVI1/FCPFrEvtBtnSyncReq ==
  FCP_FrEvt_BtnSyncReq : Inport
  UnitConverter : DataTypeConversion  OutDataTypeStr=uint8
  VHAL_FCPFrEvtBtnSyncReq_flg : Outport
  wires:
  UnitConverter/1 -> VHAL_FCPFrEvtBtnSyncReq_flg/1
  FCP_FrEvt_BtnSyncReq/1 -> UnitConverter/1

== system halin/HAL_IN/CAN2/IVI1/IVIAutoWipHSpdSWCmd ==
  IVI_AutoWipHSpdSW_Cmd : Inport
  UnitConverter : DataTypeConversion  OutDataTypeStr=uint8
  VHAL_IVIAutoWipHSpdSWCmd_flg : Outport
  wires:
  UnitConverter/1 -> VHAL_IVIAutoWipHSpdSWCmd_flg/1
  IVI_AutoWipHSpdSW_Cmd/1 -> UnitConverter/1

== system halin/HAL_IN/CAN2/IVI1/IVICreateAccReqSta ==
  IVI_CreateAccReq_Sta : Inport
  UnitConverter : DataTypeConversion  OutDataTypeStr=uint8
  VHAL_IVICreateAccReqSta_enum : Outport
  wires:
  UnitConverter/1 -> VHAL_IVICreateAccReqSta_enum/1
  IVI_CreateAccReq_Sta/1 -> UnitConverter/1

== system halin/HAL_IN/CAN2/IVI1/IVIDelAccReqSta ==
  IVI_DelAccReq_Sta : Inport
  UnitConverter : DataTypeConversion  OutDataTypeStr=uint8
  VHAL_IVIDelAccReqSta_enum : Outport
  wires:
  UnitConverter/1 -> VHAL_IVIDelAccReqSta_enum/1
  IVI_DelAccReq_Sta/1 -> UnitConverter/1

== system halin/HAL_IN/CAN2/IVI1/IVIDrivingLockSWSta ==
  IVI_Driving_Lock_SW_Sta : Inport
  UnitConverter : DataTypeConversion  OutDataTypeStr=uint8
  VHAL_IVIDrivingLockSWSta_flg : Outport
  wires:
  UnitConverter/1 -> VHAL_IVIDrivingLockSWSta_flg/1
  IVI_Driving_Lock_SW_Sta/1 -> UnitConverter/1

== system halin/HAL_IN/CAN2/IVI1/IVIFrTrunkUnlockReqSta ==
  IVI_FrTrunk_UnlockReq_Sta : Inport
  UnitConverter : DataTypeConversion  OutDataTypeStr=uint8
  VHAL_IVIFrTrunkUnlockReqSta_flg : Outport
  wires:
  UnitConverter/1 -> VHAL_IVIFrTrunkUnlockReqSta_flg/1
  IVI_FrTrunk_UnlockReq_Sta/1 -> UnitConverter/1

== system halin/HAL_IN/CAN2/IVI1/IVILinkAccReqSta ==
  IVI_LinkAccReq_Sta : Inport
  UnitConverter : DataTypeConversion  OutDataTypeStr=uint8
  VHAL_IVILinkAccReqSta_flg : Outport
  wires:
  UnitConverter/1 -> VHAL_IVILinkAccReqSta_flg/1
  IVI_LinkAccReq_Sta/1 -> UnitConverter/1

== system halin/HAL_IN/CAN2/IVI1/IVILinkAccSta ==
  IVI_LinkAcc_Sta : Inport
  UnitConverter : DataTypeConversion  OutDataTypeStr=uint8
  VHAL_IVILinkAccSta_enum : Outport
  wires:
  UnitConverter/1 -> VHAL_IVILinkAccSta_enum/1
  IVI_LinkAcc_Sta/1 -> UnitConverter/1

== system halin/HAL_IN/CAN2/IVI1/IVILinkKeySta ==
  IVI_LinkKey_Sta : Inport
  UnitConverter : DataTypeConversion  OutDataTypeStr=uint8
  VHAL_IVILinkKeySta_enum : Outport
  wires:
  UnitConverter/1 -> VHAL_IVILinkKeySta_enum/1
  IVI_LinkKey_Sta/1 -> UnitConverter/1

== system halin/HAL_IN/CAN2/IVI1/IVILocatedSTA ==
  IVI_Located_STA : Inport
  UnitConverter : DataTypeConversion  OutDataTypeStr=uint8
  VHAL_IVILocatedSTA_enum : Outport
  wires:
  UnitConverter/1 -> VHAL_IVILocatedSTA_enum/1
  IVI_Located_STA/1 -> UnitConverter/1

== system halin/HAL_IN/CAN2/IVI1/IVILockSoundSWSta ==
  IVI_Lock_SoundSW_Sta : Inport
  UnitConverter : DataTypeConversion  OutDataTypeStr=uint8
  VHAL_IVILockSoundSWSta_flg : Outport
  wires:
  UnitConverter/1 -> VHAL_IVILockSoundSWSta_flg/1
  IVI_Lock_SoundSW_Sta/1 -> UnitConverter/1

== system halin/HAL_IN/CAN2/IVI1/IVIQuickRefreshSta ==
  IVI_QuickRefresh_Sta : Inport
  UnitConverter : DataTypeConversion  OutDataTypeStr=uint8
  VHAL_IVIQuickRefreshSta_flg : Outport
  wires:
  UnitConverter/1 -> VHAL_IVIQuickRefreshSta_flg/1
  IVI_QuickRefresh_Sta/1 -> UnitConverter/1

== system halin/HAL_IN/CAN2/IVI1/IVISWCVibModeSta ==
  IVI_SWC_VibMode_Sta : Inport
  UnitConverter : DataTypeConversion  OutDataTypeStr=uint8
  VHAL_IVISWCVibModeSta_enum : Outport
  wires:
  UnitConverter/1 -> VHAL_IVISWCVibModeSta_enum/1
  IVI_SWC_VibMode_Sta/1 -> UnitConverter/1

== system halin/HAL_IN/CAN2/IVI1/IVIStoppingUnlockSWSta ==
  IVI_Stopping_Unlock_SW_Sta : Inport
  UnitConverter : DataTypeConversion  OutDataTypeStr=uint8
  VHAL_IVIStoppingUnlockSWSta_flg : Outport
  wires:
  UnitConverter/1 -> VHAL_IVIStoppingUnlockSWSta_flg/1
  IVI_Stopping_Unlock_SW_Sta/1 -> UnitConverter/1

== system halin/HAL_IN/CAN2/IVI1/IVITimeCheck ==
  IVI_Time_Check : Inport
  UnitConverter : DataTypeConversion  OutDataTypeStr=uint8
  VHAL_IVITimeCheck_enum : Outport
  wires:
  UnitConverter/1 -> VHAL_IVITimeCheck_enum/1
  IVI_Time_Check/1 -> UnitConverter/1

== system halin/HAL_IN/CAN2/IVI1/IVITimeDay ==
  IVI_Time_Day : Inport
  UnitConverter : DataTypeConversion  OutDataTypeStr=uint8
  VHAL_IVITimeDay_DAY : Outport
  wires:
  UnitConverter/1 -> VHAL_IVITimeDay_DAY/1
  IVI_Time_Day/1 -> UnitConverter/1

== system halin/HAL_IN/CAN2/IVI1/IVITimeHour ==
  IVI_Time_Hour : Inport
  UnitConverter : DataTypeConversion  OutDataTypeStr=uint8
  VHAL_IVITimeHour_hr : Outport
  wires:
  UnitConverter/1 -> VHAL_IVITimeHour_hr/1
  IVI_Time_Hour/1 -> UnitConverter/1

== system halin/HAL_IN/CAN2/IVI1/IVITimeMinute ==
  IVI_Time_Minute : Inport
  UnitConverter : DataTypeConversion  OutDataTypeStr=uint8
  VHAL_IVITimeMinute_min : Outport
  wires:
  UnitConverter/1 -> VHAL_IVITimeMinute_min/1
  IVI_Time_Minute/1 -> UnitConverter/1

== system halin/HAL_IN/CAN2/IVI1/IVITimeMonth ==
  IVI_Time_Month : Inport
  UnitConverter : DataTypeConversion  OutDataTypeStr=uint8
  VHAL_IVITimeMonth_MONTH : Outport
  wires:
  UnitConverter/1 -> VHAL_IVITimeMonth_MONTH/1
  IVI_Time_Month/1 -> UnitConverter/1

== system halin/HAL_IN/CAN2/IVI1/IVITimeSecond ==
  IVI_Time_Second : Inport
  UnitConverter : DataTypeConversion  OutDataTypeStr=uint8
  VHAL_IVITimeSecond_s : Outport
  wires:
  UnitConverter/1 -> VHAL_IVITimeSecond_s/1
  IVI_Time_Second/1 -> UnitConverter/1

== system halin/HAL_IN/CAN2/IVI1/IVITimeYear ==
  IVI_Time_Year : Inport
  UnitConverter : DataTypeConversion  OutDataTypeStr=uint8
  convert_in : FVT_lib/hal/convert_in  gain=1  offset=2000
  VHAL_IVITimeYear_YEAR : Outport
  wires:
  convert_in/1 -> VHAL_IVITimeYear_YEAR/1
  UnitConverter/1 -> convert_in/1
  IVI_Time_Year/1 -> UnitConverter/1

== system halin/HAL_IN/CAN2/IVI1/IVIWPTCSWSta ==
  IVI_WPTC_SW_Sta : Inport
  UnitConverter : DataTypeConversion  OutDataTypeStr=uint8
  VHAL_IVIWPTCSWSta_flg : Outport
  wires:
  UnitConverter/1 -> VHAL_IVIWPTCSWSta_flg/1
  IVI_WPTC_SW_Sta/1 -> UnitConverter/1

== system halin/HAL_IN/CAN2/IVI1/IVIsigScreenReqSta ==
  IVI_sigScreenReq_Sta : Inport
  UnitConverter : DataTypeConversion  OutDataTypeStr=uint8
  VHAL_IVIsigScreenReqSta_flg : Outport
  wires:
  UnitConverter/1 -> VHAL_IVIsigScreenReqSta_flg/1
  IVI_sigScreenReq_Sta/1 -> UnitConverter/1

== system halin/HAL_IN/CAN2/IVI1/LINKtoDrive ==
  LINKtoDrive : Inport
  UnitConverter : DataTypeConversion  OutDataTypeStr=uint8
  VHAL_LINKtoDrive_flg : Outport
  wires:
  UnitConverter/1 -> VHAL_LINKtoDrive_flg/1
  LINKtoDrive/1 -> UnitConverter/1

== system halin/HAL_IN/CAN2/IVI1/OpenDrOpenWdoSW ==
  OpenDrOpenWdo_SW : Inport
  UnitConverter : DataTypeConversion  OutDataTypeStr=uint8
  VHAL_OpenDrOpenWdoSW_flg : Outport
  wires:
  UnitConverter/1 -> VHAL_OpenDrOpenWdoSW_flg/1
  OpenDrOpenWdo_SW/1 -> UnitConverter/1

== system halin/HAL_IN/CAN2/IVI1/PWCONTINUEUSE ==
  PW_CONTINUE_USE : Inport
  UnitConverter : DataTypeConversion  OutDataTypeStr=uint8
  VHAL_PWCONTINUEUSE_flg : Outport
  wires:
  UnitConverter/1 -> VHAL_PWCONTINUEUSE_flg/1
  PW_CONTINUE_USE/1 -> UnitConverter/1

== system halin/HAL_IN/CAN2/IVI1/SmartEcoModeSW ==
  SmartEco_Mode_SW : Inport
  UnitConverter : DataTypeConversion  OutDataTypeStr=uint8
  VHAL_SmartEcoModeSW_flg : Outport
  wires:
  UnitConverter/1 -> VHAL_SmartEcoModeSW_flg/1
  SmartEco_Mode_SW/1 -> UnitConverter/1

== system halin/HAL_IN/CAN2/IVI1/UserSet ==
  UserSet : Inport
  UnitConverter : DataTypeConversion  OutDataTypeStr=uint8
  VHAL_UserSet_enum : Outport
  wires:
  UnitConverter/1 -> VHAL_UserSet_enum/1
  UserSet/1 -> UnitConverter/1

== system halin/HAL_IN/CAN2/IVI2/ACChgCurSet ==
  AC_Chg_Cur_Set : Inport
  UnitConverter : DataTypeConversion  OutDataTypeStr=uint8
  convert_in : FVT_lib/hal/convert_in  gain=1  offset=5
  VHAL_ACChgCurSet_A : Outport
  wires:
  convert_in/1 -> VHAL_ACChgCurSet_A/1
  UnitConverter/1 -> convert_in/1
  AC_Chg_Cur_Set/1 -> UnitConverter/1

== system halin/HAL_IN/CAN2/IVI2/AVMErrSTA ==
  AVM_Err_STA : Inport
  UnitConverter : DataTypeConversion  OutDataTypeStr=uint8
  VHAL_AVMErrSTA_flg : Outport
  wires:
  UnitConverter/1 -> VHAL_AVMErrSTA_flg/1
  AVM_Err_STA/1 -> UnitConverter/1

== system halin/HAL_IN/CAN2/IVI2/AVMOFFRecButt ==
  AVM_OFF_Rec_Butt : Inport
  UnitConverter : DataTypeConversion  OutDataTypeStr=uint8
  VHAL_AVMOFFRecButt_flg : Outport
  wires:
  UnitConverter/1 -> VHAL_AVMOFFRecButt_flg/1
  AVM_OFF_Rec_Butt/1 -> UnitConverter/1

== system halin/HAL_IN/CAN2/IVI2/AVMParkingmode ==
  AVM_Parking_mode : Inport
  UnitConverter : DataTypeConversion  OutDataTypeStr=uint8
  VHAL_AVMParkingmode_enum : Outport
  wires:
  UnitConverter/1 -> VHAL_AVMParkingmode_enum/1
  AVM_Parking_mode/1 -> UnitConverter/1

== system halin/HAL_IN/CAN2/IVI2/AVMparkingcancel ==
  AVM_parking_cancel : Inport
  UnitConverter : DataTypeConversion  OutDataTypeStr=uint8
  VHAL_AVMparkingcancel_enum : Outport
  wires:
  UnitConverter/1 -> VHAL_AVMparkingcancel_enum/1
  AVM_parking_cancel/1 -> UnitConverter/1

== system halin/HAL_IN/CAN2/IVI2/AVMparkingexcute ==
  AVM_parking_excute : Inport
  UnitConverter : DataTypeConversion  OutDataTypeStr=uint8
  VHAL_AVMparkingexcute_enum : Outport
  wires:
  UnitConverter/1 -> VHAL_AVMparkingexcute_enum/1
  AVM_parking_excute/1 -> UnitConverter/1

== system halin/HAL_IN/CAN2/IVI2/ApproachUnlockSW ==
  Approach_Unlock_SW : Inport
  UnitConverter : DataTypeConversion  OutDataTypeStr=uint8
  VHAL_ApproachUnlockSW_flg : Outport
  wires:
  UnitConverter/1 -> VHAL_ApproachUnlockSW_flg/1
  Approach_Unlock_SW/1 -> UnitConverter/1

== system halin/HAL_IN/CAN2/IVI2/CAASSw ==
  CAAS_Sw : Inport
  UnitConverter : DataTypeConversion  OutDataTypeStr=uint8
  VHAL_CAASSw_enum : Outport
  wires:
  UnitConverter/1 -> VHAL_CAASSw_enum/1
  CAAS_Sw/1 -> UnitConverter/1

== system halin/HAL_IN/CAN2/IVI2/CDLLockButt ==
  CDL_Lock_Butt : Inport
  UnitConverter : DataTypeConversion  OutDataTypeStr=uint8
  VHAL_CDLLockButt_flg : Outport
  wires:
  UnitConverter/1 -> VHAL_CDLLockButt_flg/1
  CDL_Lock_Butt/1 -> UnitConverter/1

== system halin/HAL_IN/CAN2/IVI2/CDLUnlockButt ==
  CDL_Unlock_Butt : Inport
  UnitConverter : DataTypeConversion  OutDataTypeStr=uint8
  VHAL_CDLUnlockButt_flg : Outport
  wires:
  UnitConverter/1 -> VHAL_CDLUnlockButt_flg/1
  CDL_Unlock_Butt/1 -> UnitConverter/1

== system halin/HAL_IN/CAN2/IVI2/DSEATantiset ==
  DSEAT_anti_set : Inport
  UnitConverter : DataTypeConversion  OutDataTypeStr=uint8
  VHAL_DSEATantiset_flg : Outport
  wires:
  UnitConverter/1 -> VHAL_DSEATantiset_flg/1
  DSEAT_anti_set/1 -> UnitConverter/1

== system halin/HAL_IN/CAN2/IVI2/DSEATentryfunset ==
  DSEAT_entryfun_set : Inport
  UnitConverter : DataTypeConversion  OutDataTypeStr=uint8
  VHAL_DSEATentryfunset_flg : Outport
  wires:
  UnitConverter/1 -> VHAL_DSEATentryfunset_flg/1
  DSEAT_entryfun_set/1 -> UnitConverter/1

== system halin/HAL_IN/CAN2/IVI2/DSEATventreq ==
  DSEAT_vent_req : Inport
  UnitConverter : DataTypeConversion  OutDataTypeStr=uint8
  VHAL_DSEATventreq_enum : Outport
  wires:
  UnitConverter/1 -> VHAL_DSEATventreq_enum/1
  DSEAT_vent_req/1 -> UnitConverter/1

== system halin/HAL_IN/CAN2/IVI2/Distanceunit ==
  Distance_unit : Inport
  UnitConverter : DataTypeConversion  OutDataTypeStr=uint8
  VHAL_Distanceunit_flg : Outport
  wires:
  UnitConverter/1 -> VHAL_Distanceunit_flg/1
  Distance_unit/1 -> UnitConverter/1

== system halin/HAL_IN/CAN2/IVI2/ESCSWCmd ==
  ESC_SW_Cmd : Inport
  UnitConverter : DataTypeConversion  OutDataTypeStr=uint8
  VHAL_ESCSWCmd_enum : Outport
  wires:
  UnitConverter/1 -> VHAL_ESCSWCmd_enum/1
  ESC_SW_Cmd/1 -> UnitConverter/1

== system halin/HAL_IN/CAN2/IVI2/FSOffSw ==
  FS_Off_Sw : Inport
  UnitConverter : DataTypeConversion  OutDataTypeStr=uint8
  VHAL_FSOffSw_enum : Outport
  wires:
  UnitConverter/1 -> VHAL_FSOffSw_enum/1
  FS_Off_Sw/1 -> UnitConverter/1

== system halin/HAL_IN/CAN2/IVI2/FollowMeSW ==
  FollowMeSW : Inport
  UnitConverter : DataTypeConversion  OutDataTypeStr=uint8
  VHAL_FollowMeSW_flg : Outport
  wires:
  UnitConverter/1 -> VHAL_FollowMeSW_flg/1
  FollowMeSW/1 -> UnitConverter/1

== system halin/HAL_IN/CAN2/IVI2/GPSLAT ==
  GPS_LAT : Inport
  UnitConverter : DataTypeConversion  OutDataTypeStr=uint32
  VHAL_GPSLAT_s : Outport
  wires:
  UnitConverter/1 -> VHAL_GPSLAT_s/1
  GPS_LAT/1 -> UnitConverter/1

== system halin/HAL_IN/CAN2/IVI2/GPSLONG ==
  GPS_LONG : Inport
  UnitConverter : DataTypeConversion  OutDataTypeStr=uint32
  VHAL_GPSLONG_enum : Outport
  wires:
  UnitConverter/1 -> VHAL_GPSLONG_enum/1
  GPS_LONG/1 -> UnitConverter/1

== system halin/HAL_IN/CAN2/IVI2/HeadLampSW ==
  HeadLampSW : Inport
  UnitConverter : DataTypeConversion  OutDataTypeStr=uint8
  VHAL_HeadLampSW_enum : Outport
  wires:
  UnitConverter/1 -> VHAL_HeadLampSW_enum/1
  HeadLampSW/1 -> UnitConverter/1

== system halin/HAL_IN/CAN2/IVI2/HoodLatchSW ==
  Hood_Latch_SW : Inport
  UnitConverter : DataTypeConversion  OutDataTypeStr=uint8
  VHAL_HoodLatchSW_enum : Outport
  wires:
  UnitConverter/1 -> VHAL_HoodLatchSW_enum/1
  Hood_Latch_SW/1 -> UnitConverter/1

== system halin/HAL_IN/CAN2/IVI2/IVIACCAdaptiveSta ==
  IVI_ACC_Adaptive_Sta : Inport
  UnitConverter : DataTypeConversion  OutDataTypeStr=uint8
  VHAL_IVIACCAdaptiveSta_flg : Outport
  wires:
  UnitConverter/1 -> VHAL_IVIACCAdaptiveSta_flg/1
  IVI_ACC_Adaptive_Sta/1 -> UnitConverter/1

== system halin/HAL_IN/CAN2/IVI2/IVIAirIntZ3Cmd ==
  IVI_AirIntZ3_Cmd : Inport
  UnitConverter : DataTypeConversion  OutDataTypeStr=uint8
  VHAL_IVIAirIntZ3Cmd_enum : Outport
  wires:
  UnitConverter/1 -> VHAL_IVIAirIntZ3Cmd_enum/1
  IVI_AirIntZ3_Cmd/1 -> UnitConverter/1

== system halin/HAL_IN/CAN2/IVI2/IVIChargePortSWSta ==
  IVI_ChargePortSW_Sta : Inport
  UnitConverter : DataTypeConversion  OutDataTypeStr=uint8
  VHAL_IVIChargePortSWSta_flg : Outport
  wires:
  UnitConverter/1 -> VHAL_IVIChargePortSWSta_flg/1
  IVI_ChargePortSW_Sta/1 -> UnitConverter/1

== system halin/HAL_IN/CAN2/IVI2/IVICreepSWReq ==
  IVI_CreepSW_Req : Inport
  UnitConverter : DataTypeConversion  OutDataTypeStr=uint8
  VHAL_IVICreepSWReq_flg : Outport
  wires:
  UnitConverter/1 -> VHAL_IVICreepSWReq_flg/1
  IVI_CreepSW_Req/1 -> UnitConverter/1

== system halin/HAL_IN/CAN2/IVI2/IVIDSEATFroEdgeHeightCmd ==
  IVI_DSEAT_FroEdge_Height_Cmd : Inport
  UnitConverter : DataTypeConversion  OutDataTypeStr=uint8
  VHAL_IVIDSEATFroEdgeHeightCmd_enum : Outport
  wires:
  UnitConverter/1 -> VHAL_IVIDSEATFroEdgeHeightCmd_enum/1
  IVI_DSEAT_FroEdge_Height_Cmd/1 -> UnitConverter/1

== system halin/HAL_IN/CAN2/IVI2/IVIDSEATHeaterCmd ==
  IVI_DSEATHeater_Cmd : Inport
  UnitConverter : DataTypeConversion  OutDataTypeStr=uint8
  VHAL_IVIDSEATHeaterCmd_enum : Outport
  wires:
  UnitConverter/1 -> VHAL_IVIDSEATHeaterCmd_enum/1
  IVI_DSEATHeater_Cmd/1 -> UnitConverter/1

== system halin/HAL_IN/CAN2/IVI2/IVIDSEATHeightCmd ==
  IVI_DSEAT_Height_Cmd : Inport
  UnitConverter : DataTypeConversion  OutDataTypeStr=uint8
  VHAL_IVIDSEATHeightCmd_enum : Outport
  wires:
  UnitConverter/1 -> VHAL_IVIDSEATHeightCmd_enum/1
  IVI_DSEAT_Height_Cmd/1 -> UnitConverter/1

== system halin/HAL_IN/CAN2/IVI2/IVIDSEATMemory1Sta ==
  IVI_DSEAT_Memory1_Sta : Inport
  UnitConverter : DataTypeConversion  OutDataTypeStr=uint8
  VHAL_IVIDSEATMemory1Sta_flg : Outport
  wires:
  UnitConverter/1 -> VHAL_IVIDSEATMemory1Sta_flg/1
  IVI_DSEAT_Memory1_Sta/1 -> UnitConverter/1

== system halin/HAL_IN/CAN2/IVI2/IVIDSEATMemory2Sta ==
  IVI_DSEAT_Memory2_Sta : Inport
  UnitConverter : DataTypeConversion  OutDataTypeStr=uint8
  VHAL_IVIDSEATMemory2Sta_flg : Outport
  wires:
  UnitConverter/1 -> VHAL_IVIDSEATMemory2Sta_flg/1
  IVI_DSEAT_Memory2_Sta/1 -> UnitConverter/1

== system halin/HAL_IN/CAN2/IVI2/IVIDSEATMemoryOPTCLSSta ==
  IVI_DSEAT_Memory_OPTCLS_Sta : Inport
  UnitConverter : DataTypeConversion  OutDataTypeStr=uint8
  VHAL_IVIDSEATMemoryOPTCLSSta_flg : Outport
  wires:
  UnitConverter/1 -> VHAL_IVIDSEATMemoryOPTCLSSta_flg/1
  IVI_DSEAT_Memory_OPTCLS_Sta/1 -> UnitConverter/1

== system halin/HAL_IN/CAN2/IVI2/IVIDSEATReclineCmd ==
  IVI_DSEAT_Recline_Cmd : Inport
  UnitConverter : DataTypeConversion  OutDataTypeStr=uint8
  VHAL_IVIDSEATReclineCmd_enum : Outport
  wires:
  UnitConverter/1 -> VHAL_IVIDSEATReclineCmd_enum/1
  IVI_DSEAT_Recline_Cmd/1 -> UnitConverter/1

== system halin/HAL_IN/CAN2/IVI2/IVIDSEATSlideCmd ==
  IVI_DSEAT_Slide_Cmd : Inport
  UnitConverter : DataTypeConversion  OutDataTypeStr=uint8
  VHAL_IVIDSEATSlideCmd_enum : Outport
  wires:
  UnitConverter/1 -> VHAL_IVIDSEATSlideCmd_enum/1
  IVI_DSEAT_Slide_Cmd/1 -> UnitConverter/1

== system halin/HAL_IN/CAN2/IVI2/IVIFGSAirIntCmd ==
  IVI_FGSAirInt_Cmd : Inport
  UnitConverter : DataTypeConversion  OutDataTypeStr=uint8
  VHAL_IVIFGSAirIntCmd_enum : Outport
  wires:
  UnitConverter/1 -> VHAL_IVIFGSAirIntCmd_enum/1
  IVI_FGSAirInt_Cmd/1 -> UnitConverter/1

== system halin/HAL_IN/CAN2/IVI2/IVIFGSChCmd ==
  IVI_FGSCh_Cmd : Inport
  UnitConverter : DataTypeConversion  OutDataTypeStr=uint8
  VHAL_IVIFGSChCmd_enum : Outport
  wires:
  UnitConverter/1 -> VHAL_IVIFGSChCmd_enum/1
  IVI_FGSCh_Cmd/1 -> UnitConverter/1

== system halin/HAL_IN/CAN2/IVI2/IVIIONSWCmd ==
  IVI_IONSW_Cmd : Inport
  UnitConverter : DataTypeConversion  OutDataTypeStr=uint8
  VHAL_IVIIONSWCmd_flg : Outport
  wires:
  UnitConverter/1 -> VHAL_IVIIONSWCmd_flg/1
  IVI_IONSW_Cmd/1 -> UnitConverter/1

== system halin/HAL_IN/CAN2/IVI2/IVIISAOffsetSpd ==
  IVI_ISA_OffsetSpd : Inport
  UnitConverter : DataTypeConversion  OutDataTypeStr=uint8
  VHAL_IVIISAOffsetSpd_enum : Outport
  wires:
  UnitConverter/1 -> VHAL_IVIISAOffsetSpd_enum/1
  IVI_ISA_OffsetSpd/1 -> UnitConverter/1

== system halin/HAL_IN/CAN2/IVI2/IVINightModeSta ==
  IVI_Night_Mode_Sta : Inport
  UnitConverter : DataTypeConversion  OutDataTypeStr=uint8
  VHAL_IVINightModeSta_flg : Outport
  wires:
  UnitConverter/1 -> VHAL_IVINightModeSta_flg/1
  IVI_Night_Mode_Sta/1 -> UnitConverter/1

== system halin/HAL_IN/CAN2/IVI2/IVIPSEATHeaterCmd ==
  IVI_PSEATHeater_Cmd : Inport
  UnitConverter : DataTypeConversion  OutDataTypeStr=uint8
  VHAL_IVIPSEATHeaterCmd_enum : Outport
  wires:
  UnitConverter/1 -> VHAL_IVIPSEATHeaterCmd_enum/1
  IVI_PSEATHeater_Cmd/1 -> UnitConverter/1

== system halin/HAL_IN/CAN2/IVI2/IVIPSEATReclineCmd ==
  IVI_PSEAT_Recline_Cmd : Inport
  UnitConverter : DataTypeConversion  OutDataTypeStr=uint8
  VHAL_IVIPSEATReclineCmd_enum : Outport
  wires:
  UnitConverter/1 -> VHAL_IVIPSEATReclineCmd_enum/1
  IVI_PSEAT_Recline_Cmd/1 -> UnitConverter/1
